simulink model "b"  (R2023a)
settings: Solver=VariableStepAuto  StartTime=0.0  StopTime=10.0  RelTol=1e-3
settings Model: Creator=eriknymobohne  LastModifiedBy=eriknymobohne

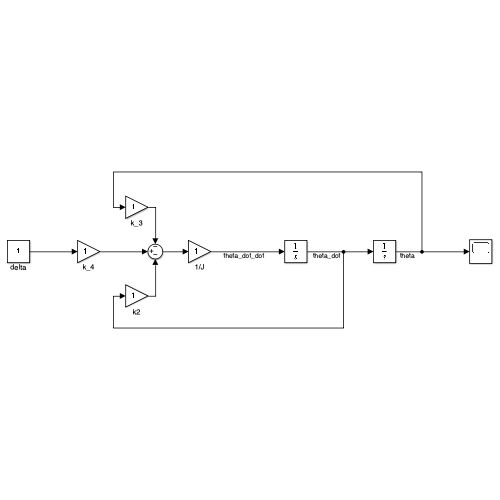
[thumbnail: Simulink's stored preview of the top-level diagram]
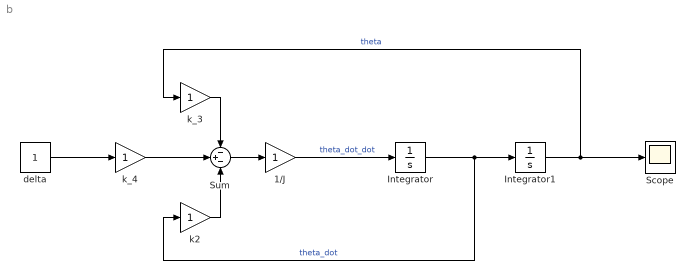
== system b ==
  1/J : Gain
  Integrator : Integrator
  Integrator1 : Integrator
  Scope : Scope
  Sum : Sum  Inputs=-+-
  delta : Constant
  k2 : Gain
  k_3 : Gain
  k_4 : Gain
  wires:
  delta/1 -> k_4/1
  Sum/1 -> 1/J/1
  Integrator/1 -> k2/1, Integrator1/1  "theta_dot"
  Integrator1/1 -> k_3/1, Scope/1  "theta"
  k_4/1 -> Sum/2
  k_3/1 -> Sum/1
  k2/1 -> Sum/3
  1/J/1 -> Integrator/1  "theta_dot_dot"
